simulink model "fm_mod_demod_simulink"  (R2018a)
settings: Solver=VariableStepAuto  StartTime=0.0  StopTime=10.0  RelTol=1e-3
libraries: commanabbnd3 x2
settings Model: Creator=Hassan  LastModifiedBy=Hassan

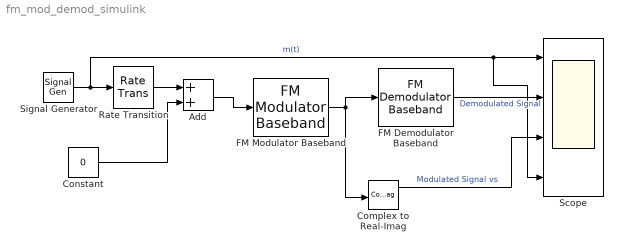
== system fm_mod_demod_simulink ==
  "Add " : Sum
  "Complex to Real-Imag " : ComplexToRealImag
  "Constant " : Constant  Value=0
  "FM Demodulator Baseband " : commanabbnd3/FM Demodulator Baseband   FrequencyDeviation=100  SimulateUsing=Code generation
      settings: SourceProductName=Communications System Toolbox  SourceProductBaseCode=CM
  "FM Modulator Baseband " : commanabbnd3/FM Modulator Baseband  FrequencyDeviation=100  SimulateUsing=Code generation
      settings: SourceProductName=Communications System Toolbox  SourceProductBaseCode=CM
  "Rate Transition " : RateTransition  OutPortSampleTime=1/100e3
  Scope : Scope  NumInputPorts=4
  "Signal Generator " : SignalGenerator  Frequency=5  Units=rad/sec
  wires:
  "Rate Transition "/1 -> "Add "/1
  "Constant "/1 -> "Add "/2
  "Signal Generator "/1 -> Scope/4, Scope/1, "Rate Transition "/1  "m(t)"
  "Add "/1 -> "FM Modulator Baseband "/1
  "FM Modulator Baseband "/1 -> "FM Demodulator Baseband "/1, "Complex to Real-Imag "/1
  "Complex to Real-Imag "/1 -> Scope/3  "Modulated Signal vs"
  "FM Demodulator Baseband "/1 -> Scope/2  "Demodulated Signal"
